simulink model "LaserPropulsion_v1_0"  (R2016a)
settings: Solver=ode45  StartTime=0.0  StopTime=1000  RelTol=1e-3
undefined symbols (not defined in the file): Cm
libraries: simulink x1
settings Model: Creator=sakshi  LastModifiedBy=sakshi

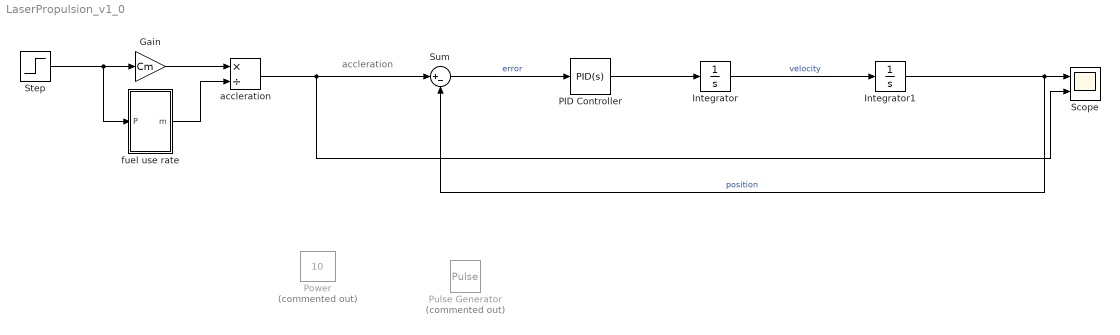
== system LaserPropulsion_v1_0 ==
  note: accleration
  Gain : Gain  Gain=Cm
  Integrator : Integrator  InitialCondition=1  ZeroCross=off
  Integrator1 : Integrator  InitialCondition=1  ZeroCross=off
  PID Controller : simulink/Continuous/PID Controller  Controller=PID  TimeDomain=Continuous-time  SampleTime=-1  IntegratorMethod=Forward Euler  FilterMethod=Forward Euler  Form=Parallel  UseFilter=on  ControllerParametersSource=internal  P=0.18567926327114  I=0.00869253354119013  D=0.973920981598194  N=5.45397025421619  InitialConditionSource=internal  InitialConditionForIntegrator=0  InitialConditionForFilter=0  ExternalReset=none  LimitOutput=off  UpperSaturationLimit=inf  LowerSaturationLimit=-inf  LinearizeAsGain=on  AntiWindupMode=none  Kb=1  TrackingMode=off  Kt=1  PParamMin=[]  PParamMax=[]  IParamMin=[]  IParamMax=[]  DParamMin=[]  DParamMax=[]  NParamMin=[]  NParamMax=[]  KbParamMin=[]  KbParamMax=[]  KtParamMin=[]  KtParamMax=[]  POutMin=[]  POutMax=[]  IOutMin=[]  IOutMax=[]  DOutMin=[]  DOutMax=[]  NOutMin=[]  NOutMax=[]  KbOutMin=[]  KbOutMax=[]  KtOutMin=[]  KtOutMax=[]  IntegratorOutMin=[]  IntegratorOutMax=[]  FilterOutMin=[]  FilterOutMax=[]  SumOutMin=[]  SumOutMax=[]  SumI1OutMin=[]  SumI1OutMax=[]  SumI2OutMin=[]  SumI2OutMax=[]  SumI3OutMin=[]  SumI3OutMax=[]  SumDOutMin=[]  SumDOutMax=[]  SaturationOutMin=[]  SaturationOutMax=[]  IntegratorContinuousStateAttributes=''  IntegratorStateMustResolveToSignalObject=off  IntegratorRTWStateStorageClass=Auto  FilterContinuousStateAttributes=''  FilterStateMustResolveToSignalObject=off  FilterRTWStateStorageClass=Auto  DifferentiatorICPrevScaledInput=0  DifferentiatorOutMin=[]  DifferentiatorOutMax=[]
  Power : Constant  Commented=on  Value=10
  Pulse Generator : DiscretePulseGenerator  Commented=on  PulseType=Time based  Period=10  PulseWidth=5
  Scope : Scope  NumInputPorts=2
  Step : Step  SampleTime=0
  Sum : Sum  Inputs=|+-
  accleration : Product  Inputs=*/
  "fuel use rate " : Subsystem
  wires:
  Integrator/1 -> Integrator1/1  "velocity"
  Integrator1/1 -> Sum/2, Scope/1  "position"
  Sum/1 -> PID Controller/1  "error"
  Step/1 -> "fuel use rate "/1("P "), Gain/1
  Gain/1 -> accleration/1
  accleration/1 -> Sum/1, Scope/2
  PID Controller/1 -> Integrator/1
  "fuel use rate "/1("m ") -> accleration/2

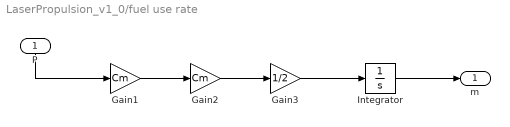
== system LaserPropulsion_v1_0/fuel use rate  ==
  "P " : Inport
  Gain1 : Gain  Gain=Cm
  Gain2 : Gain  Gain=Cm
  Gain3 : Gain  Gain=1/2
  Integrator : Integrator  InitialCondition=1  ZeroCross=off
  "m " : Outport
  wires:
  Gain2/1 -> Gain3/1
  "P "/1 -> Gain1/1
  Gain1/1 -> Gain2/1
  Gain3/1 -> Integrator/1
  Integrator/1 -> "m "/1
